simulink model "Laengsdynamik"  (R2019a)
settings: Solver=ode4  StartTime=0.0  StopTime=10.0  FixedStep=0.001  RelTol=1e-3
model workspace (MAT data in the model file):
  FBv = [-0.360628002737 -0.359628002737 -0.358628002737 -0.357628002737 -0.356628002737 -0.355628002737 -0.354628002737 -0.353628002737 -0.352628002737 -0.351628002737 -0.350628002737 -0.349628002737 ... (3119 elements, 1x3119)]
  G_g = 16.59
  G_h = 8.17
  g = 9.81
  h_s = 0.5
  l = 2.8
  l_v = 1.344
  reifenX = [0 0.25 1]
  reifenY = [0 1 1]
  useController = 1
  v0 = 22.2222222222
  z_time = [0 1.5 1.95 2.15 10]
  z_vals = [0 0 0.1 1 1]
  zh_z = 1
  zv_z = 1
libraries: simulink x3
(part 1 of 2)
settings Model: Creator=phlippe  LastModifiedBy=Mel
settings DataIOCC: ReturnWorkspaceOutputs=off
settings DebuggingCC: ArithmeticOperatorsInVariantConditions=warning
settings SFSimCC: SimUseLocalCustomCode=off
settings RTWCC: RTWUseLocalCustomCode=off

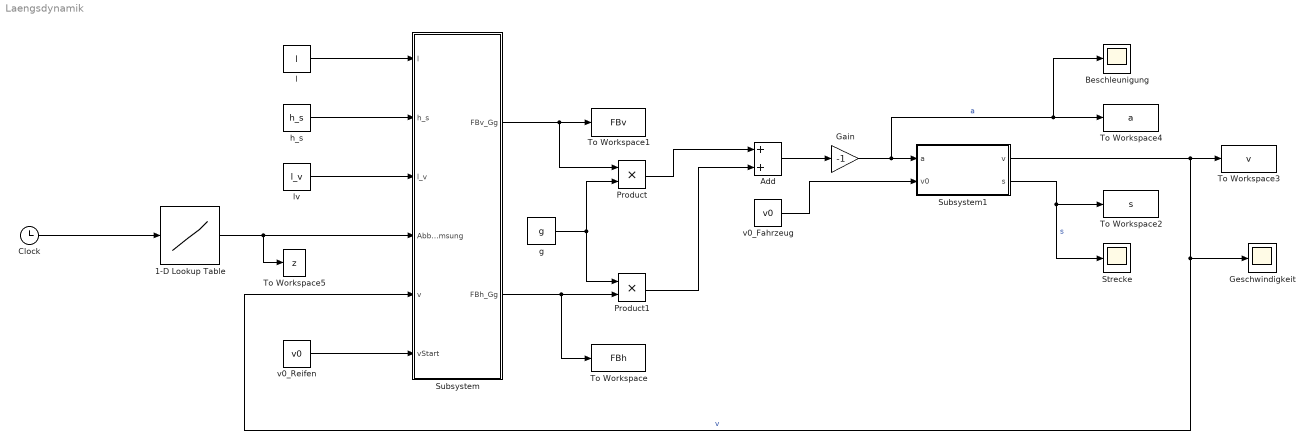
== system Laengsdynamik ==
  1-D Lookup Table : Lookup_n-D  NumberOfTableDimensions=1  BreakpointsForDimension1=z_time  Table=z_vals  ExtrapMethod=Clip  UseLastTableValue=on  InternalRulePriority=Speed  RndMeth=Simplest  InputSameDT=on
  Add : Sum
  Beschleunigung : Scope
  Clock : Clock
  Gain : Gain  Gain=-1
  Geschwindigkeit : Scope
  Product : Product
  Product1 : Product
  Strecke : Scope
  Subsystem : Subsystem
  Subsystem1 : Subsystem
  To Workspace : ToWorkspace  VariableName=FBh  SaveFormat=Timeseries  SampleTime=-1
  To Workspace1 : ToWorkspace  VariableName=FBv  SaveFormat=Timeseries  SampleTime=-1
  To Workspace2 : ToWorkspace  VariableName=s  SaveFormat=Timeseries  SampleTime=-1
  To Workspace3 : ToWorkspace  VariableName=v  SaveFormat=Timeseries  SampleTime=-1
  To Workspace4 : ToWorkspace  VariableName=a  SaveFormat=Timeseries  SampleTime=-1
  To Workspace5 : ToWorkspace  VariableName=z  SaveFormat=Timeseries  SampleTime=-1
  "g " : Constant  Value=g
  h_s : Constant  Value=h_s
  l : Constant  Value=l
  "lv " : Constant  Value=l_v
  v0_Fahrzeug : Constant  Value=v0
  v0_Reifen : Constant  Value=v0
  wires:
  h_s/1 -> Subsystem/2(h_s)
  l/1 -> Subsystem/1(l)
  "lv "/1 -> Subsystem/3(l_v)
  1-D Lookup Table/1 -> Subsystem/4(Abbremsung), To Workspace5/1
  Clock/1 -> 1-D Lookup Table/1
  Subsystem/1(FBv_Gg) -> Product/1, To Workspace1/1
  "g "/1 -> Product/2, Product1/1
  Product/1 -> Add/1
  Product1/1 -> Add/2
  Add/1 -> Gain/1
  v0_Fahrzeug/1 -> Subsystem1/2("v0 ")
  Gain/1 -> Beschleunigung/1, To Workspace4/1, Subsystem1/1(a)  "a"
  Subsystem1/2(s) -> Strecke/1, To Workspace2/1  "s"
  Subsystem1/1(v) -> Geschwindigkeit/1, Subsystem/5(v), To Workspace3/1  "v"
  Subsystem/2(FBh_Gg) -> To Workspace/1, Product1/2
  v0_Reifen/1 -> Subsystem/6(vStart)

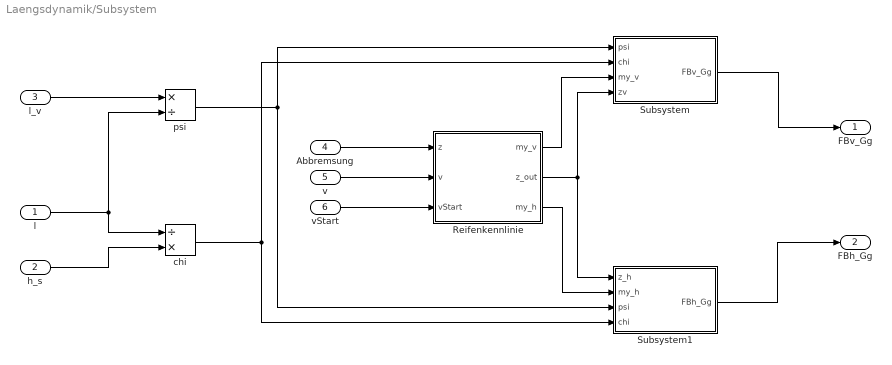
== system Laengsdynamik/Subsystem ==
  l : Inport
  h_s : Inport  Port=2
  l_v : Inport  Port=3
  Abbremsung : Inport  Port=4
  v : Inport  Port=5
  vStart : Inport  Port=6
  Reifenkennlinie : Subsystem
  Subsystem : Subsystem
  Subsystem1 : Subsystem
  chi : Product  Inputs=/*
  "psi " : Product  Inputs=*/
  FBv_Gg : Outport
  FBh_Gg : Outport  Port=2
  wires:
  h_s/1 -> chi/2
  l/1 -> chi/1, "psi "/2
  l_v/1 -> "psi "/1
  Subsystem/1(FBv_Gg) -> FBv_Gg/1
  "psi "/1 -> Subsystem/1(psi), Subsystem1/3(psi)
  chi/1 -> Subsystem1/4(chi), Subsystem/2(chi)
  Subsystem1/1(FBh_Gg) -> FBh_Gg/1
  v/1 -> Reifenkennlinie/2(v)
  Abbremsung/1 -> Reifenkennlinie/1(z)
  Reifenkennlinie/1(my_v) -> Subsystem/3(my_v)
  Reifenkennlinie/2(z_out) -> Subsystem1/1(z_h), Subsystem/4(zv)
  Reifenkennlinie/3(my_h) -> Subsystem1/2(my_h)
  vStart/1 -> Reifenkennlinie/3(vStart)

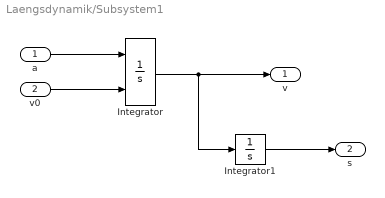
== system Laengsdynamik/Subsystem1 ==
  a : Inport
  "v0 " : Inport  Port=2
  Integrator : Integrator  InitialConditionSource=external  LimitOutput=on  LowerSaturationLimit=0
  Integrator1 : Integrator
  v : Outport
  s : Outport  Port=2
  wires:
  a/1 -> Integrator/1
  "v0 "/1 -> Integrator/2
  Integrator/1 -> Integrator1/1, v/1
  Integrator1/1 -> s/1
